simulink library "LIB_TF_G_12_StepControl"  (Simulink 8.6)
settings: Solver=ode45  StartTime=0.0  StopTime=10.0  RelTol=1e-3
PreLoadFcn:
  | if exist('tl_preloadfcn','file'), tl_preloadfcn(gcs,402); end
PostLoadFcn:
  | if exist('tl_postloadfcn','file'), tl_postloadfcn(gcs,402); end
undefined symbols (not defined in the file): ddv, u2, u3
libraries: tllib x4, LIB_TF_G_12_StepControl x1
(part 7 of 7)

== stateflow chart TF_G_12_ControlStepExecution/ChartManageLatencyTimer ==
  settings: description=$TL$ name=$O; stepfunctionclass=STATIC_FCN_ASR4; functionname=$O; $TL$
  (default) -> (junction 20)
  (junction 20) -> (junction 21) [order 1] : /* Check the Null Power of Motor */
      | [ (lNextConsign == KL_ZERO) || bPreviousIsStepFrozen == KB_TRUE ]
  (junction 21) -> (junction 22)
  (junction 20) -> (junction 24) [order 2] : /* Make a Backup of the last non null order sign */
      | {
      | cPreviousSign = cSign;
      | }
  (junction 22) -> (junction 23) [order 1] : [ cPreviousMotorPowerOrder != int8(KUC_ZERO) ]
  (junction 22) -> (junction 26) [order 2]
  (junction 23) -> (junction 27) : {
      | usCounter = uint16(0);
      | }
  (junction 24) -> (junction 25) [order 1] : [ lNextConsign > KL_ZERO ]
  (junction 24) -> (junction 28) [order 2] : /* The Sign is negativ */
      | {
      | cSign = int8(int8(KUC_ZERO) - int8(KUC_ONE));
      | }
  (junction 25) -> (junction 29) : /* The sign is positiv */
      | {
      | cSign = int8(KUC_ONE);
      | }
  (junction 26) -> (junction 27) [order 1] : /* Check the upper limit */
      | [usCounter >= KUS_LATENCY_TIME]
  (junction 26) -> (junction 34) [order 2] : /* Increment counter */
      | {
      | usCounter = usCounter + KUS_STEP_SELECTION_PERIOD;
      | }
  (junction 27) -> (junction 35)
  (junction 29) -> (junction 28)
  (junction 28) -> (junction 30)
  (junction 30) -> (junction 31) [order 1] : [ cSign == cPreviousSign ]
  (junction 30) -> (junction 32) [order 2] : /* Increment counter */
      | {usCounter = usCounter + KUS_STEP_SELECTION_PERIOD;}
  (junction 31) -> (junction 33) : /* Reset Counter */
      | {usCounter = uint16(0) ;}
  (junction 33) -> (junction 32)
  (junction 34) -> (junction 33)
  (junction 35) -> (junction 34)
  (junction 32) -> (junction 36)
  (junction 36) -> (junction 37) [order 1] : [ (int8(cSign*cPreviousSign) == int8(int8(KUC_ZERO)-int8(KUC_ONE))) && ...
      | usCounter < KUS_LATENCY_TIME ]
  (junction 36) -> (junction 38) [order 2] : {
      | bIsStepFrozen = KB_FALSE;
      | }
  (junction 37) -> (junction 39) : {
      | bIsStepFrozen = KB_TRUE;
      | }
  (junction 39) -> (junction 38)
  (junction 38) -> (junction 40)
  data: bPreviousIsStepFrozen input double; cPreviousMotorPowerOrder input int8 =0; lNextConsign input double; bIsStepFrozen output boolean =0; KB_FALSE constant uint8 =ddv('BFE/KB_FALSE'); KB_TRUE constant uint8 =ddv('BFE/KB_TRUE'); KC_ZERO constant int8 =ddv('Common/KS8_ZERO'); cPreviousSign local int8 =0; cSign local int8 =0; usCounter local uint16 size=1 [0..255] =0; KUC_ONE constant uint8 =ddv('Common/KU8_ONE'); KUS_LATENCY_TIME constant uint16 =ddv('BFE_Config_Data/KUS_LATENCY_TIME'); KUS_STEP_SELECTION_PERIOD constant uint16 =ddv('Sampling_Freq/KUS_STEP_SELECTION_PERIOD'); KS_ZERO constant int16 =ddv('Common/KS16_ZERO'); usPreviousCounter local uint16 =0; KL_ZERO constant int32 =ddv('Common/KS32_ZERO'); KUC_ZERO constant uint8 =ddv('Common/KU8_ZERO')
  data bPreviousIsStepFrozen settings: description=$TL$ type=Bool; $TL$
  data cPreviousMotorPowerOrder settings: description=$TL$ type=Int8; $TL$
  data lNextConsign settings: description=$TL$ type=Int32; $TL$
  data bIsStepFrozen settings: description=$TL$ name=$O; type=Bool; $TL$
  data KB_FALSE settings: description=$TL$ variable=BFE/KB_FALSE; $TL$
  data KB_TRUE settings: description=$TL$ variable=BFE/KB_TRUE; $TL$
  data KC_ZERO settings: description=$TL$ variable=Common/KS8_ZERO; $TL$
  data cPreviousSign settings: description=$TL$ type=Int8; $TL$
  data cSign settings: description=$TL$ type=Int8; $TL$
  data usCounter settings: description=$TL$ type=UInt16; $TL$
  data KUC_ONE settings: description=$TL$ variable=Common/KU8_ONE; $TL$
  data KUS_LATENCY_TIME settings: description=$TL$ variable=BFE_Config_Data/KUS_LATENCY_TIME; $TL$
  data KUS_STEP_SELECTION_PERIOD settings: description=$TL$ variable=Sampling_Freq/KUS_STEP_SELECTION_PERIOD; $TL$
  data KS_ZERO settings: description=$TL$ variable=Common/KS16_ZERO; $TL$
  data usPreviousCounter settings: description=$TL$ type=UInt16; $TL$
  data KL_ZERO settings: description=$TL$ variable=Common/KS32_ZERO; $TL$
  data KUC_ZERO settings: description=$TL$ variable=Common/KU8_ZERO; $TL$
